simulink model "IFOR"  (Simulink 7.1)
settings: Solver=ode1  StartTime=0  StopTime=1  FixedStep=1e-5  MaxStep=1e-4  RelTol=1e-3  AbsTol=1e-6
undefined symbols (not defined in the file): I1, I2, I3, ids, Lm, P, P1, P2, P3, Rr, Rs, Tr, Ud, wb, Xlr, Xls, Xm
libraries: simulink x3
settings Model: Creator=Karsten  LastModifiedBy=Karsten  ExtModeTrigMode=oneshot  ExtModeArmWhenConnect=off
settings SolverCC: InitialStep=1e-4
settings DataIOCC: LimitDataPoints=off  SignalLoggingName=sigsOut
settings OptimizationCC: BooleanDataType=off  InlineInvariantSignals=on
settings DebuggingCC: SaveWithParameterizedLinksMsg=none  CheckExecutionContextPreStartOutputMsg=on  CheckExecutionContextRuntimeOutputMsg=on  SignalResolutionControl=TryResolveAllWithWarning  SolverPrmCheckMsg=none  MultiTaskDSMMsg=warning  MultiTaskCondExecSysMsg=none  StrictBusMsg=None
settings HardwareCC: TargetUnknown=on
settings RTWCC: TemplateMakefile=grt_vc.tmf  IncludeERTFirstTime=on
settings GRTTargetCC: TargetFcnLib=ansi_tfl_tmw.mat

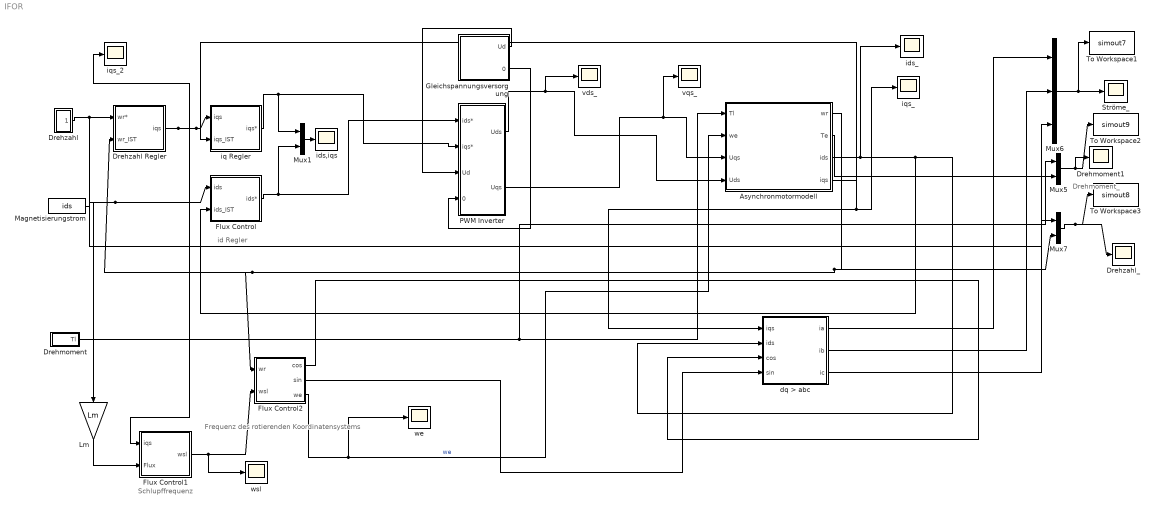
== system IFOR ==
  note: Schlupffrequenz
  note: Frequenz des rotierenden
      | Koordinatensystems
  note: id Regler
  note: Drehmoment_
  Asynchronmotormodell : Subsystem
  Drehmoment : Subsystem
  Drehmoment1 : Scope
      settings: TickLabels=on  TimeRange=0.001543443952852636  YMin=-3  YMax=6  DataFormat=Array  MaxDataPoints=500000
  Drehzahl : Subsystem
  Drehzahl Regler : Subsystem
  Drehzahl_ : Scope
      settings: TickLabels=on  TimeRange=0.5  YMin=156.4  YMax=157.1  DataFormat=Array  MaxDataPoints=500000
  Flux Control : Subsystem
  Flux Control1 : Subsystem
  Flux Control2 : Subsystem
  Gleichspannungsversorgung : Subsystem
  Lm : Gain  Orientation=down  Gain=Lm  ParameterDataType=sfix(16)  ParameterScaling=2^0  OutDataType=sfix(16)  OutScaling=2^0
  Magnetisierungstrom : Constant  Value=ids  OutDataType=sfix(16)  OutScaling=2^0
  Mux1 : Mux  Inputs=2
  Mux5 : Mux  Inputs=2
  Mux6 : Mux  Inputs=3
  Mux7 : Mux  Inputs=2
  PWM Inverter : Subsystem
  Ströme_ : Scope
      settings: TickLabels=on  TimeRange=0.008485639686684032  YMin=-4  YMax=4  DataFormat=Array  MaxDataPoints=500000
  To Workspace1 : ToWorkspace  VariableName=simout7  SampleTime=-1  SaveFormat=Structure
  To Workspace2 : ToWorkspace  VariableName=simout9  SampleTime=-1  SaveFormat=Structure
  To Workspace3 : ToWorkspace  VariableName=simout8  SampleTime=-1  SaveFormat=Structure
  dq > abc : Subsystem
  ids,iqs : Scope
      settings: TickLabels=on  TimeRange=0.5  YMin=-0.25  YMax=3  SaveName=ScopeData8  DataFormat=Array  MaxDataPoints=500000
  ids_ : Scope
      settings: TickLabels=on  TimeRange=0.3  YMin=0.65  YMax=0.8300000000000001  SaveName=ScopeData17  DataFormat=Array  MaxDataPoints=500000
  iq Regler : Subsystem
  iqs_ : Scope
      settings: TickLabels=on  TimeRange=0.3  YMin=3.15  YMax=3.8  SaveName=ScopeData18  DataFormat=Array  MaxDataPoints=500000
  iqs_2 : Scope
      settings: TickLabels=on  TimeRange=0.3  YMin=-1  YMax=-0.1  SaveName=ScopeData9  DataFormat=Array  MaxDataPoints=500000
  vds_ : Scope
      settings: TickLabels=on  TimeRange=0.3  YMin=-150  YMax=150  SaveName=ScopeData20  DataFormat=Array  MaxDataPoints=500000
  vqs_ : Scope
      settings: TickLabels=on  TimeRange=0.3  YMin=-200  YMax=200  SaveName=ScopeData19  DataFormat=Array  MaxDataPoints=500000
  we : Scope
      settings: TickLabels=on  YMin=31.4298  YMax=31.4301  SaveName=ScopeData3  DataFormat=Array  MaxDataPoints=500000
  wsl : Scope
      settings: TickLabels=on  TimeRange=0.5  YMin=-0.0225  YMax=0.0325  SaveName=ScopeData21  DataFormat=Array  MaxDataPoints=500000
  wires:
  Drehzahl/1(wr*) -> Drehzahl Regler/1(wr*), Mux7/1
  Flux Control2/3(we) -> we/1, Asynchronmotormodell/2(we)  "we"
  Mux6/1 -> Ströme_/1, To Workspace1/1
  Mux5/1 -> Drehmoment1/1, To Workspace2/1
  Mux7/1 -> Drehzahl_/1, To Workspace3/1
  PWM Inverter/2(Uqs) -> Asynchronmotormodell/3(Uqs), vqs_/1
  Asynchronmotormodell/4(iqs) -> dq > abc/1(iqs), iqs_/1, iq Regler/2(iqs_IST)
  Asynchronmotormodell/3(ids) -> ids_/1, dq > abc/2(ids), Flux Control/2(ids_IST)
  PWM Inverter/1(Uds) -> vds_/1, Asynchronmotormodell/4(Uds)
  Drehmoment/1(Tl) -> Asynchronmotormodell/1(Tl), Mux5/1
  Asynchronmotormodell/1(wr) -> Mux7/2, Drehzahl Regler/2(wr_IST), Flux Control2/1(wr)
  Asynchronmotormodell/2(Te) -> Mux5/2
  dq > abc/1(ia) -> Mux6/1
  dq > abc/2(ib) -> Mux6/2
  dq > abc/3(ic) -> Mux6/3
  iq Regler/1(iqs*) -> Mux1/1, PWM Inverter/2(iqs*)
  Drehzahl Regler/1(iqs) -> iq Regler/1(iqs), Flux Control1/1(iqs), iqs_2/1
  Flux Control/1(ids*) -> Mux1/2, PWM Inverter/1(ids*)
  Flux Control1/1(wsl) -> Flux Control2/2(wsl), wsl/1
  Flux Control2/1(cos) -> dq > abc/3(cos)
  Flux Control2/2(sin) -> dq > abc/4(sin)
  Magnetisierungstrom/1 -> Flux Control/1(ids), Lm/1
  Lm/1 -> Flux Control1/2(Flux)
  Gleichspannungsversorgung/2(0) -> PWM Inverter/4(0)
  Gleichspannungsversorgung/1(Ud) -> PWM Inverter/3(Ud)
  Mux1/1 -> ids,iqs/1

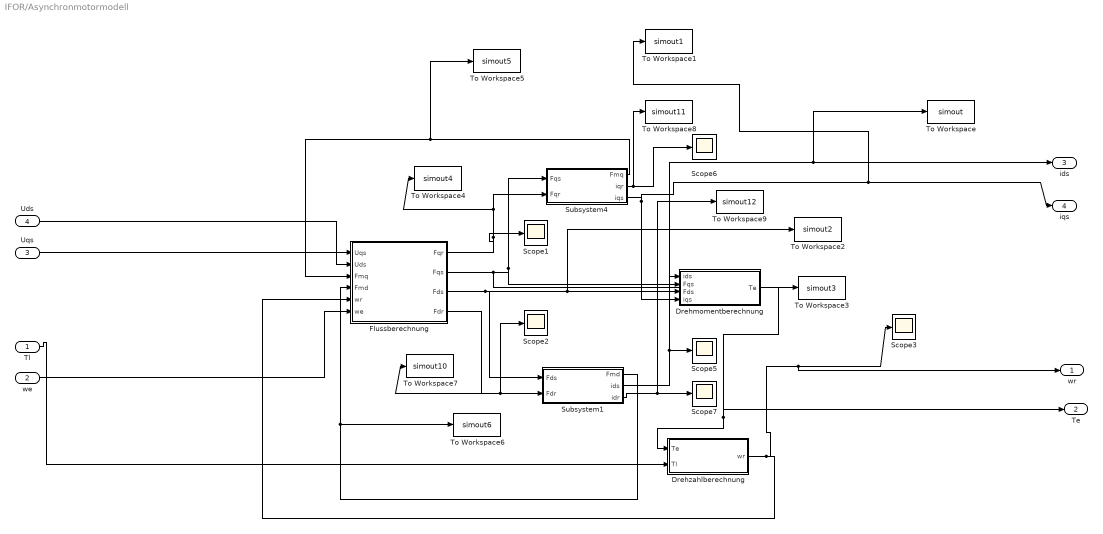
== system IFOR/Asynchronmotormodell ==
  Tl : Inport  OutDataType=sfix(16)  OutScaling=2^0
  we : Inport  Port=2  OutDataType=sfix(16)  OutScaling=2^0
  Uqs : Inport  Port=3  OutDataType=sfix(16)  OutScaling=2^0
  Uds : Inport  Port=4  OutDataType=sfix(16)  OutScaling=2^0
  Drehmomentberechnung : Subsystem
  Drehzahlberechnung : Subsystem
  Flussberechnung : Subsystem
  Scope{1..3,5..7} (6 alike) : Scope
      Scope1 settings: TimeRange=0.3  YMin=-47.25  YMax=-43.75  SaveName=ScopeData29
      Scope2 settings: TimeRange=0.3  YMin=386.5  YMax=393.5  SaveName=ScopeData30
      Scope3 settings: TimeRange=0.5  YMin=30  YMax=240  SaveName=Drehzahl1
      Scope5 settings: TimeRange=0.5  YMin=66.3  YMax=68.1  SaveName=ScopeData13
      Scope6 settings: TimeRange=0.3  YMin=-25  YMax=7.5  SaveName=ScopeData14
      Scope7 settings: TimeRange=1  YMin=-1  YMax=1  SaveName=ScopeData15
  Subsystem1 : Subsystem
  Subsystem4 : Subsystem
  To Workspace : ToWorkspace  VariableName=simout  SampleTime=-1  SaveFormat=Structure
  To Workspace1 : ToWorkspace  VariableName=simout1  SampleTime=-1  SaveFormat=Structure
  To Workspace2 : ToWorkspace  VariableName=simout2  SampleTime=-1  SaveFormat=Structure
  To Workspace3 : ToWorkspace  VariableName=simout3  SampleTime=-1  SaveFormat=Structure
  To Workspace4 : ToWorkspace  VariableName=simout4  SampleTime=-1  SaveFormat=Structure
  To Workspace5 : ToWorkspace  VariableName=simout5  SampleTime=-1  SaveFormat=Structure
  To Workspace6 : ToWorkspace  VariableName=simout6  SampleTime=-1  SaveFormat=Structure
  To Workspace7 : ToWorkspace  VariableName=simout10  SampleTime=-1  SaveFormat=Structure
  To Workspace8 : ToWorkspace  VariableName=simout11  SampleTime=-1  SaveFormat=Structure
  To Workspace9 : ToWorkspace  VariableName=simout12  SampleTime=-1  SaveFormat=Structure
  wr : Outport  OutDataType=sfix(16)  OutScaling=2^0
  Te : Outport  Port=2  OutDataType=sfix(16)  OutScaling=2^0
  ids : Outport  Port=3  OutDataType=sfix(16)  OutScaling=2^0
  iqs : Outport  Port=4  OutDataType=sfix(16)  OutScaling=2^0
  wires:
  Flussberechnung/1(Fqr) -> Subsystem4/2(Fqr), To Workspace4/1, Scope1/1
  Flussberechnung/2(Fqs) -> Subsystem4/1(Fqs), Drehmomentberechnung/2(Fqs), To Workspace3/1
  Subsystem4/1(Fmq) -> Flussberechnung/3(Fmq), To Workspace5/1
  Flussberechnung/3(Fds) -> Subsystem1/1(Fds), Drehmomentberechnung/3(Fds), To Workspace2/1
  Flussberechnung/4(Fdr) -> To Workspace7/1, Scope2/1, Subsystem1/2(Fdr)
  Subsystem1/1(Fmd) -> Flussberechnung/4(Fmd), To Workspace6/1
  Subsystem1/2(ids) -> Drehmomentberechnung/1(ids), Scope5/1, ids/1, To Workspace/1
  Subsystem1/3(idr) -> Scope7/1, To Workspace9/1
  Subsystem4/3(iqs) -> Drehmomentberechnung/4(iqs), iqs/1, To Workspace1/1
  Drehmomentberechnung/1(Te) -> Drehzahlberechnung/1(Te), Te/1
  Drehzahlberechnung/1(wr) -> Flussberechnung/5(wr), Scope3/1, wr/1
  Tl/1 -> Drehzahlberechnung/2(Tl)
  Subsystem4/2(iqr) -> Scope6/1, To Workspace8/1
  we/1 -> Flussberechnung/6(we)
  Uqs/1 -> Flussberechnung/1(Uqs)
  Uds/1 -> Flussberechnung/2(Uds)

== system IFOR/Drehmoment ==
  Step2 : Step  Time=.2  After=3  SampleTime=0
  Step3 : Step  Time=0.05  After=0  SampleTime=0
  Step4 : Step  Time=30  After=0  SampleTime=0
  Sum1 : Sum  Inputs=|+++  OutDataType=sfix(16)  OutScaling=2^0  SaturateOnIntegerOverflow=on  InputSameDT=on  OutDataTypeStr=Inherit: Same as first input
  Tl : Outport  OutDataType=sfix(16)  OutScaling=2^0
  wires:
  Step3/1 -> Sum1/2
  Step2/1 -> Sum1/1
  Step4/1 -> Sum1/3
  Sum1/1 -> Tl/1

== system IFOR/Drehzahl ==
  Magnetisierungstrom : Constant  Value=wb/5  OutDataType=sfix(16)  OutScaling=2^0
  Repeating Sequence : simulink/Sources/Repeating Sequence  SystemSampleTime=-1  rep_seq_t=[0 .15 .25 .4 .55 .6 10]  rep_seq_y=[0 .5*wb .5*wb .2*wb .2*wb .4*wb .2*wb]
  Repeating Sequence1 : simulink/Sources/Repeating Sequence  SystemSampleTime=-1  rep_seq_t=[0 .15 .25 .4 .55 .6 10]  rep_seq_y=[0 .5*wb .5*wb .5*wb .5*wb .2*wb .2*wb]
  wr* : Outport  OutDataType=sfix(16)  OutScaling=2^0
  wires:
  Repeating Sequence1/1 -> wr*/1

== system IFOR/Drehzahl Regler ==
  wr* : Inport  OutDataType=sfix(16)  OutScaling=2^0
  wr_IST : Inport  Port=2  OutDataType=sfix(16)  OutScaling=2^0
  Gain1 : Gain  Gain=P1  ParameterDataType=sfix(16)  ParameterScaling=2^0  OutDataType=sfix(16)  OutScaling=2^0
  Gain2 : Gain  Gain=I1  ParameterDataType=sfix(16)  ParameterScaling=2^0  OutDataType=sfix(16)  OutScaling=2^0
  Integrator : Integrator
  Sum4 : Sum  Inputs=|++  OutDataType=sfix(16)  OutScaling=2^0
  Sum5 : Sum  Inputs=|+-  OutDataType=sfix(16)  OutScaling=2^0
  ia4 : Scope
      settings: TickLabels=on  YMin=2675  YMax=3100  SaveName=ScopeData5  DataFormat=Array  MaxDataPoints=500000
  iqs : Outport  OutDataType=sfix(16)  OutScaling=2^0  InitialOutput=0
  wires:
  wr*/1 -> Sum5/1
  Integrator/1 -> Sum4/2
  Gain1/1 -> Sum4/1
  Gain2/1 -> Integrator/1
  Sum5/1 -> Gain1/1, Gain2/1
  wr_IST/1 -> Sum5/2
  Sum4/1 -> ia4/1, iqs/1

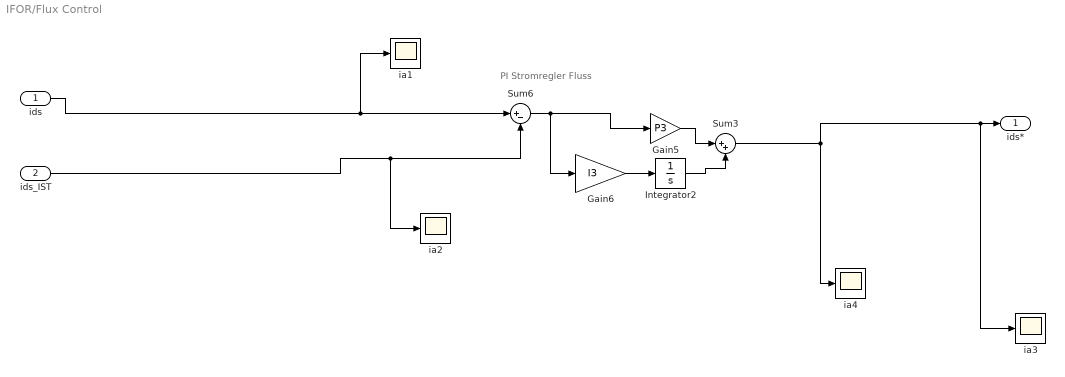
== system IFOR/Flux Control ==
  note: PI Stromregler Fluss
  ids : Inport  OutDataType=sfix(16)  OutScaling=2^0
  ids_IST : Inport  Port=2  OutDataType=sfix(16)  OutScaling=2^0
  Gain5 : Gain  Gain=P3  ParameterDataType=sfix(16)  ParameterScaling=2^0  OutDataType=sfix(16)  OutScaling=2^0
  Gain6 : Gain  Gain=I3  ParameterDataType=sfix(16)  ParameterScaling=2^0  OutDataType=sfix(16)  OutScaling=2^0
  Integrator2 : Integrator
  Sum3 : Sum  Inputs=|++  OutDataType=sfix(16)  OutScaling=2^0
  Sum6 : Sum  Inputs=|+-  OutDataType=sfix(16)  OutScaling=2^0
  ia{1..4} (4 alike) : Scope
      ia1 settings: TickLabels=on  YMin=2.3  YMax=2.3  SaveName=ScopeData24  DataFormat=Array  MaxDataPoints=500000
      ia2 settings: TickLabels=on  YMin=0.685  YMax=0.745  SaveName=ScopeData25  DataFormat=Array  MaxDataPoints=500000
      ia3 settings: TickLabels=on  YMin=-0.05  YMax=1  SaveName=ScopeData26  DataFormat=Array  MaxDataPoints=500000
      ia4 settings: TickLabels=on  YMin=-0.25  SaveName=ScopeData6  DataFormat=Array  MaxDataPoints=500000
  ids* : Outport  OutDataType=sfix(16)  OutScaling=2^0  InitialOutput=0
  wires:
  Integrator2/1 -> Sum3/2
  Gain5/1 -> Sum3/1
  Gain6/1 -> Integrator2/1
  Sum6/1 -> Gain5/1, Gain6/1
  ids_IST/1 -> Sum6/2, ia2/1
  Sum3/1 -> ia4/1, ids*/1, ia3/1
  ids/1 -> Sum6/1, ia1/1

== system IFOR/Flux Control1 ==
  iqs : Inport  OutDataType=sfix(16)  OutScaling=2^0
  Flux : Inport  Port=2  OutDataType=sfix(16)  OutScaling=2^0
  Gain : Gain  Gain=Lm/(Tr)  ParameterDataType=sfix(16)  ParameterScaling=2^0  OutDataType=sfix(16)  OutScaling=2^0  SaturateOnIntegerOverflow=on  OutDataTypeStr=Inherit: Same as input  ParamDataTypeStr=Inherit: Same as input
  Product : Product  OutDataType=sfix(16)  OutScaling=2^0  SaturateOnIntegerOverflow=on  InputSameDT=on  OutDataTypeStr=Inherit: Same as first input
  wsl : Outport  OutDataType=sfix(16)  OutScaling=2^0  InitialOutput=0
  wires:
  iqs/1 -> Gain/1
  Product/1 -> wsl/1
  Gain/1 -> Product/1
  Flux/1 -> Product/2

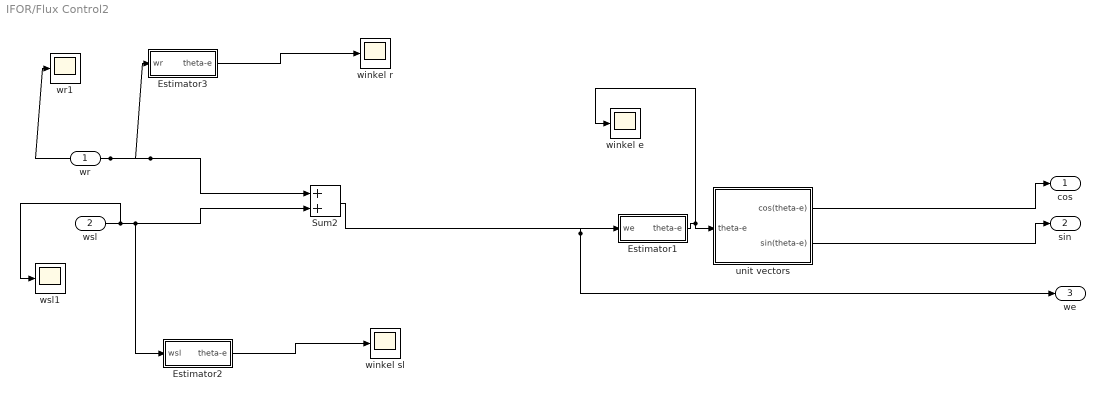
== system IFOR/Flux Control2 ==
  wr : Inport  OutDataType=sfix(16)  OutScaling=2^0
  wsl : Inport  Port=2  OutDataType=sfix(16)  OutScaling=2^0
  Estimator1 : Subsystem
  Estimator2 : Subsystem
  Estimator3 : Subsystem
  Sum2 : Sum  OutDataType=sfix(16)  OutScaling=2^0  SaturateOnIntegerOverflow=on  InputSameDT=on  OutDataTypeStr=Inherit: Same as first input
  unit vectors : Subsystem
  winkel e : Scope
      settings: TickLabels=on  YMin=0  YMax=6.5  SaveName=ScopeData4  DataFormat=Array  MaxDataPoints=500000
  winkel r : Scope
      settings: TickLabels=on  TimeRange=0.5  YMin=0  YMax=6.5  SaveName=ScopeData11  DataFormat=Array  MaxDataPoints=500000
  winkel sl : Scope
      settings: TickLabels=on  TimeRange=0.5  YMin=1.69116  YMax=1.69132  SaveName=ScopeData10  DataFormat=Array  MaxDataPoints=500000
  wr1 : Scope
      settings: TickLabels=on  YMin=156  YMax=170  SaveName=ScopeData12  DataFormat=Array  MaxDataPoints=500000
  wsl1 : Scope
      settings: TickLabels=on  YMin=-0.175  YMax=0.225  SaveName=ScopeData16  DataFormat=Array  MaxDataPoints=500000
  cos : Outport  OutDataType=sfix(16)  OutScaling=2^0  InitialOutput=0
  sin : Outport  Port=2  OutDataType=sfix(16)  OutScaling=2^0  InitialOutput=0
  we : Outport  Port=3  OutDataType=sfix(16)  OutScaling=2^0  InitialOutput=0
  wires:
  wr/1 -> Sum2/1, Estimator3/1(wr), wr1/1
  wsl/1 -> Sum2/2, Estimator2/1(wsl), wsl1/1
  unit vectors/1(cos(theta-e)) -> cos/1
  unit vectors/2(sin(theta-e)) -> sin/1
  Estimator1/1(theta-e) -> unit vectors/1(theta-e), winkel e/1
  Sum2/1 -> we/1, Estimator1/1(we)
  Estimator2/1(theta-e) -> winkel sl/1
  Estimator3/1(theta-e) -> winkel r/1

== system IFOR/Gleichspannungsversorgung ==
  Constant4 : Constant  Value=0  OutDataType=sfix(16)  OutScaling=2^0
  Constant5 : Constant  Value=Ud  OutDataType=sfix(16)  OutScaling=2^0
  Ud : Outport  OutDataType=sfix(16)  OutScaling=2^0  InitialOutput=0
  0 : Outport  Port=2  OutDataType=sfix(16)  OutScaling=2^0  InitialOutput=0
  wires:
  Constant4/1 -> 0/1
  Constant5/1 -> Ud/1

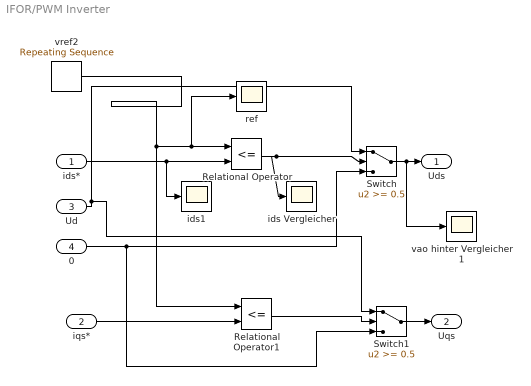
== system IFOR/PWM Inverter ==
  ids* : Inport  OutDataType=sfix(16)  OutScaling=2^0
  iqs* : Inport  Port=2  OutDataType=sfix(16)  OutScaling=2^0
  Ud : Inport  Port=3  OutDataType=sfix(16)  OutScaling=2^0
  0 : Inport  Port=4  OutDataType=sfix(16)  OutScaling=2^0
  Relational Operator : RelationalOperator  Operator=<=  InputSameDT=on
  Relational Operator1 : RelationalOperator  Operator=<=  InputSameDT=on
  Switch : Switch  Threshold=0.5  SaturateOnIntegerOverflow=on  InputSameDT=on
  Switch1 : Switch  Threshold=0.5  SaturateOnIntegerOverflow=on  InputSameDT=on
  ids Vergleicher : Scope
      settings: TickLabels=on  TimeRange=8.811583259921477e-005  YMin=-1  YMax=1  SaveName=ScopeData35  DataFormat=Array  MaxDataPoints=500000
  ids1 : Scope
      settings: TickLabels=on  TimeRange=0.3  YMin=-0.55  YMax=0.15  SaveName=ScopeData34  DataFormat=Array  MaxDataPoints=500000
  ref : Scope
      settings: TickLabels=on  TimeRange=0.3  YMin=0.9999999998750002  YMax=1.000000000125  SaveName=ScopeData33  DataFormat=Array  MaxDataPoints=500000
  vao hinter Vergleicher1 : Scope
      settings: TickLabels=on  TimeRange=0.3  YMin=-2  YMax=2  SaveName=ScopeData36  DataFormat=Array  MaxDataPoints=500000
  vref2 : simulink/Sources/Repeating Sequence  SystemSampleTime=-1  rep_seq_t=[0 25e-9 50e-9 75e-9 100e-9]  rep_seq_y=[0 1 0 -1 0]
  Uds : Outport  OutDataType=sfix(16)  OutScaling=2^0
  Uqs : Outport  Port=2  OutDataType=sfix(16)  OutScaling=2^0
  wires:
  ids*/1 -> Relational Operator/2, ids1/1
  Switch/1 -> Uds/1, vao hinter Vergleicher1/1
  Ud/1 -> Switch/1, Switch1/1
  Relational Operator/1 -> Switch/2, ids Vergleicher/1
  iqs*/1 -> Relational Operator1/2
  Switch1/1 -> Uqs/1
  Relational Operator1/1 -> Switch1/2
  vref2/1 -> Relational Operator/1, ref/1, Relational Operator1/1
  0/1 -> Switch/3, Switch1/3

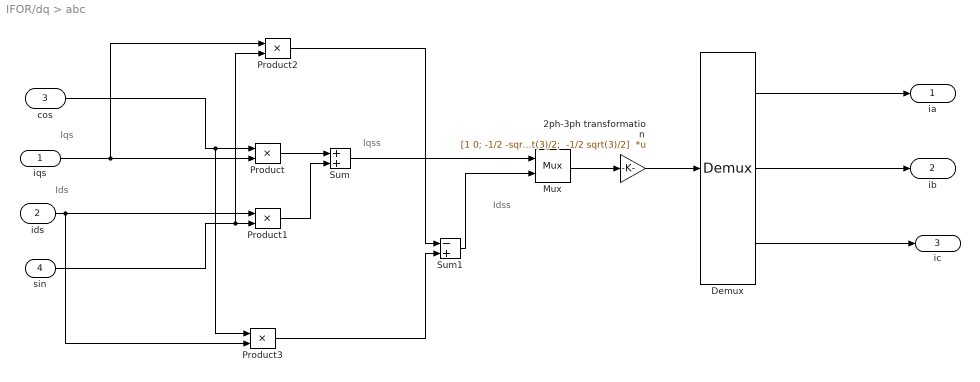
== system IFOR/dq > abc ==
  note: Ids
  note: Idss
  note: Iqs
  note: Iqss
  iqs : Inport  OutDataType=sfix(16)  OutScaling=2^0
  ids : Inport  Port=2  OutDataType=sfix(16)  OutScaling=2^0
  cos : Inport  Port=3  OutDataType=sfix(16)  OutScaling=2^0
  sin : Inport  Port=4  OutDataType=sfix(16)  OutScaling=2^0
  2ph-3ph transformation : Gain  Gain="[1 0; -1/2 -sqrt(3)/2;  -1/2 sqrt(3)/2]"  Multiplication=Matrix(K*u)  ParameterDataType=sfix(16)  ParameterScaling=2^0  OutDataType=sfix(16)  OutScaling=2^0  SaturateOnIntegerOverflow=on  OutDataTypeStr=Inherit: Same as input  ParamDataTypeStr=Inherit: Same as input
  Demux : Demux  Outputs=3
  Mux : Mux  Inputs=2
  Product{,1..3} (4 alike) : Product  OutDataType=sfix(16)  OutScaling=2^0  SaturateOnIntegerOverflow=on  InputSameDT=on  OutDataTypeStr=Inherit: Same as first input
  Sum : Sum  OutDataType=sfix(16)  OutScaling=2^0  SaturateOnIntegerOverflow=on  InputSameDT=on  OutDataTypeStr=Inherit: Same as first input
  Sum1 : Sum  Inputs=-+  OutDataType=sfix(16)  OutScaling=2^0  SaturateOnIntegerOverflow=on  InputSameDT=on  OutDataTypeStr=Inherit: Same as first input
  ia : Outport  OutDataType=sfix(16)  OutScaling=2^0
  ib : Outport  Port=2  OutDataType=sfix(16)  OutScaling=2^0
  ic : Outport  Port=3  OutDataType=sfix(16)  OutScaling=2^0
  wires:
  Demux/3 -> ic/1
  Demux/2 -> ib/1
  Demux/1 -> ia/1
  iqs/1 -> Product/2, Product2/1
  ids/1 -> Product1/1, Product3/2
  Mux/1 -> 2ph-3ph transformation/1
  Product2/1 -> Sum1/1
  Product3/1 -> Sum1/2
  cos/1 -> Product/1, Product3/1
  sin/1 -> Product1/2, Product2/2
  Product1/1 -> Sum/2
  Product/1 -> Sum/1
  Sum/1 -> Mux/1
  Sum1/1 -> Mux/2
  2ph-3ph transformation/1 -> Demux/1

== system IFOR/iq Regler ==
  note: PI Stromregler Drehmoment
  iqs : Inport  OutDataType=sfix(16)  OutScaling=2^0
  iqs_IST : Inport  Port=2  OutDataType=sfix(16)  OutScaling=2^0
  Gain3 : Gain  Gain=P2  ParameterDataType=sfix(16)  ParameterScaling=2^0  OutDataType=sfix(16)  OutScaling=2^0
  Gain4 : Gain  Gain=I2  ParameterDataType=sfix(16)  ParameterScaling=2^0  OutDataType=sfix(16)  OutScaling=2^0
  Integrator1 : Integrator
  Sum1 : Sum  Inputs=|++  OutDataType=sfix(16)  OutScaling=2^0
  Sum2 : Sum  Inputs=|+-  OutDataType=sfix(16)  OutScaling=2^0
  ia1 : Scope
      settings: TickLabels=on  YMin=-100  YMax=100  SaveName=ScopeData22  DataFormat=Array  MaxDataPoints=500000
  ia2 : Scope
      settings: TickLabels=on  YMin=-100  YMax=100  SaveName=ScopeData23  DataFormat=Array  MaxDataPoints=500000
  ia4 : Scope
      settings: TickLabels=on  YMin=0.275  YMax=0.825  SaveName=ScopeData7  DataFormat=Array  MaxDataPoints=500000
  iqs* : Outport  OutDataType=sfix(16)  OutScaling=2^0  InitialOutput=0
  wires:
  iqs_IST/1 -> Sum2/2, ia2/1
  Sum1/1 -> ia4/1, iqs*/1, ia1/1
  Sum2/1 -> Gain4/1, Gain3/1
  Gain4/1 -> Integrator1/1
  Gain3/1 -> Sum1/1
  Integrator1/1 -> Sum1/2
  iqs/1 -> Sum2/1

== system IFOR/Asynchronmotormodell/Drehmomentberechnung ==
  ids : Inport  OutDataType=sfix(16)  OutScaling=2^0
  Fqs : Inport  Port=2  OutDataType=sfix(16)  OutScaling=2^0
  Fds : Inport  Port=3  OutDataType=sfix(16)  OutScaling=2^0
  iqs : Inport  Port=4  OutDataType=sfix(16)  OutScaling=2^0
  1.5*P/(2*wb) : Gain  Gain=1.5*P/(2*wb)  ParameterDataType=sfix(16)  ParameterScaling=2^0  OutDataType=sfix(16)  OutScaling=2^0
  Add3 : Sum  Inputs=-+  OutDataType=sfix(16)  OutScaling=2^-10
  Product1 : Product  OutDataType=sfix(16)  OutScaling=2^0  RndMeth=Zero
  Product2 : Product  OutDataType=sfix(16)  OutScaling=2^0  RndMeth=Zero
  Te : Outport  OutDataType=sfix(16)  OutScaling=2^0
  wires:
  Product1/1 -> Add3/1
  Product2/1 -> Add3/2
  Add3/1 -> 1.5*P/(2*wb)/1
  1.5*P/(2*wb)/1 -> Te/1
  ids/1 -> Product1/1
  Fqs/1 -> Product1/2
  Fds/1 -> Product2/1
  iqs/1 -> Product2/2

== system IFOR/Asynchronmotormodell/Drehzahlberechnung ==
  Te : Inport  OutDataType=sfix(16)  OutScaling=2^0
  Tl : Inport  Port=2  OutDataType=sfix(16)  OutScaling=2^0
  Add3 : Sum  Inputs=+-  OutDataType=sfix(16)  OutScaling=2^-10
  Integrator : Integrator
  P/(2*J) : Gain  Gain=P/(2*0.006)  ParameterDataType=sfix(16)  ParameterScaling=2^0  OutDataType=sfix(16)  OutScaling=2^0
  wr : Outport  OutDataType=sfix(16)  OutScaling=2^0
  wires:
  Te/1 -> Add3/1
  Tl/1 -> Add3/2
  Add3/1 -> P/(2*J)/1
  P/(2*J)/1 -> Integrator/1
  Integrator/1 -> wr/1

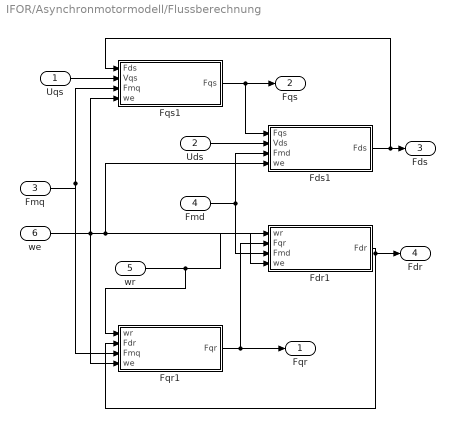
== system IFOR/Asynchronmotormodell/Flussberechnung ==
  Uqs : Inport  OutDataType=sfix(16)  OutScaling=2^0
  Uds : Inport  Port=2  OutDataType=sfix(16)  OutScaling=2^0
  Fmq : Inport  Port=3  OutDataType=sfix(16)  OutScaling=2^0
  Fmd : Inport  Port=4  OutDataType=sfix(16)  OutScaling=2^0
  wr : Inport  Port=5  OutDataType=sfix(16)  OutScaling=2^0
  we : Inport  Port=6  OutDataType=sfix(16)  OutScaling=2^0
  Fdr1 : Subsystem
  Fds1 : Subsystem
  Fqr1 : Subsystem
  Fqs1 : Subsystem
  Fqr : Outport  OutDataType=sfix(16)  OutScaling=2^0
  Fqs : Outport  Port=2  OutDataType=sfix(16)  OutScaling=2^0
  Fds : Outport  Port=3  OutDataType=sfix(16)  OutScaling=2^0
  Fdr : Outport  Port=4  OutDataType=sfix(16)  OutScaling=2^0
  wires:
  Uqs/1 -> Fqs1/2(Vqs)
  Fqs1/1(Fqs) -> Fqs/1, Fds1/1(Fqs)
  Uds/1 -> Fds1/2(Vds)
  Fmd/1 -> Fds1/3(Fmd), Fdr1/3(Fmd)
  wr/1 -> Fdr1/1(wr), Fqr1/1(wr)
  Fmq/1 -> Fqs1/3(Fmq), Fqr1/3(Fmq)
  Fdr1/1(Fdr) -> Fqr1/2(Fdr), Fdr/1
  Fqr1/1(Fqr) -> Fqr/1, Fdr1/2(Fqr)
  Fds1/1(Fds) -> Fds/1, Fqs1/1(Fds)
  we/1 -> Fqr1/4(we), Fqs1/4(we), Fdr1/4(we), Fds1/4(we)

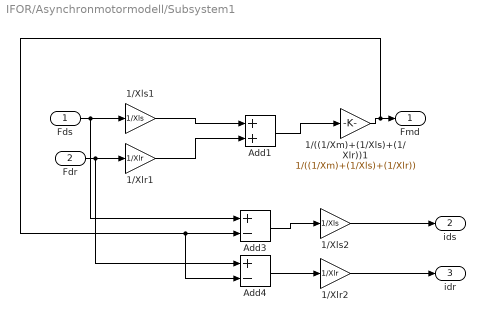
== system IFOR/Asynchronmotormodell/Subsystem1 ==
  Fds : Inport  OutDataType=sfix(16)  OutScaling=2^0
  Fdr : Inport  Port=2  OutDataType=sfix(16)  OutScaling=2^0
  1/((1/Xm)+(1/Xls)+(1/Xlr))1 : Gain  Gain=1/((1/Xm)+(1/Xls)+(1/Xlr))  ParameterDataType=sfix(16)  ParameterScaling=2^0  OutDataType=sfix(16)  OutScaling=2^0
  1/Xlr1 : Gain  Gain=1/Xlr  ParameterDataType=sfix(16)  ParameterScaling=2^0  OutDataType=sfix(16)  OutScaling=2^0
  1/Xlr2 : Gain  Gain=1/Xlr  ParameterDataType=sfix(16)  ParameterScaling=2^0  OutDataType=sfix(16)  OutScaling=2^0
  1/Xls1 : Gain  Gain=1/Xls  ParameterDataType=sfix(16)  ParameterScaling=2^0  OutDataType=sfix(16)  OutScaling=2^0
  1/Xls2 : Gain  Gain=1/Xls  ParameterDataType=sfix(16)  ParameterScaling=2^0  OutDataType=sfix(16)  OutScaling=2^0
  Add1 : Sum  OutDataType=sfix(16)  OutScaling=2^-10
  Add3 : Sum  Inputs=+-  OutDataType=sfix(16)  OutScaling=2^-10
  Add4 : Sum  Inputs=+-  OutDataType=sfix(16)  OutScaling=2^-10
  Fmd : Outport  OutDataType=sfix(16)  OutScaling=2^0
  ids : Outport  Port=2  OutDataType=sfix(16)  OutScaling=2^0
  idr : Outport  Port=3  OutDataType=sfix(16)  OutScaling=2^0
  wires:
  Fds/1 -> 1/Xls1/1, Add3/1
  Fdr/1 -> 1/Xlr1/1, Add4/1
  1/Xls1/1 -> Add1/1
  1/Xlr1/1 -> Add1/2
  Add1/1 -> 1/((1/Xm)+(1/Xls)+(1/Xlr))1/1
  1/((1/Xm)+(1/Xls)+(1/Xlr))1/1 -> Fmd/1, Add3/2, Add4/2
  Add3/1 -> 1/Xls2/1
  Add4/1 -> 1/Xlr2/1
  1/Xlr2/1 -> idr/1
  1/Xls2/1 -> ids/1

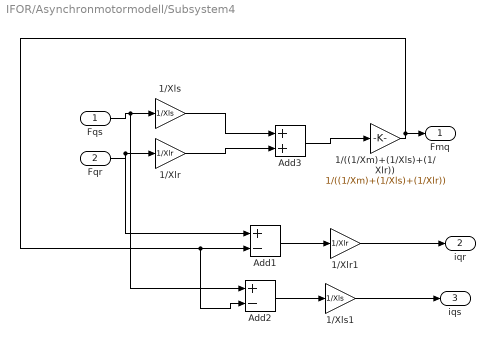
== system IFOR/Asynchronmotormodell/Subsystem4 ==
  Fqs : Inport  OutDataType=sfix(16)  OutScaling=2^0
  Fqr : Inport  Port=2  OutDataType=sfix(16)  OutScaling=2^0
  1/((1/Xm)+(1/Xls)+(1/Xlr)) : Gain  Gain=1/((1/Xm)+(1/Xls)+(1/Xlr))  ParameterDataType=sfix(16)  ParameterScaling=2^0  OutDataType=sfix(16)  OutScaling=2^0
  1/Xlr : Gain  Gain=1/Xlr  ParameterDataType=sfix(16)  ParameterScaling=2^0  OutDataType=sfix(16)  OutScaling=2^0
  1/Xlr1 : Gain  Gain=1/Xlr  ParameterDataType=sfix(16)  ParameterScaling=2^0  OutDataType=sfix(16)  OutScaling=2^0
  1/Xls : Gain  Gain=1/Xls  ParameterDataType=sfix(16)  ParameterScaling=2^0  OutDataType=sfix(16)  OutScaling=2^0
  1/Xls1 : Gain  Gain=1/Xls  ParameterDataType=sfix(16)  ParameterScaling=2^0  OutDataType=sfix(16)  OutScaling=2^0
  Add1 : Sum  Inputs=+-  OutDataType=sfix(16)  OutScaling=2^-10
  Add2 : Sum  Inputs=+-  OutDataType=sfix(16)  OutScaling=2^-10
  Add3 : Sum  OutDataType=sfix(16)  OutScaling=2^-10
  Fmq : Outport  OutDataType=sfix(16)  OutScaling=2^0
  iqr : Outport  Port=2  OutDataType=sfix(16)  OutScaling=2^0
  iqs : Outport  Port=3  OutDataType=sfix(16)  OutScaling=2^0
  wires:
  Fqs/1 -> 1/Xls/1, Add2/1
  Fqr/1 -> 1/Xlr/1, Add1/1
  1/Xls/1 -> Add3/1
  1/Xlr/1 -> Add3/2
  Add3/1 -> 1/((1/Xm)+(1/Xls)+(1/Xlr))/1
  1/((1/Xm)+(1/Xls)+(1/Xlr))/1 -> Fmq/1, Add1/2, Add2/2
  Add1/1 -> 1/Xlr1/1
  1/Xlr1/1 -> iqr/1
  Add2/1 -> 1/Xls1/1
  1/Xls1/1 -> iqs/1

== system IFOR/Flux Control2/Estimator1 ==
  we : Inport  OutDataType=sfix(16)  OutScaling=2^0
  Constant : Constant  Value=2*pi  OutDataType=sfix(16)  OutScaling=2^0
  Integrator : Integrator  InitialCondition=pi/6
  Math Function3 : Math  Operator=mod  OutDataType=sfix(16)  OutScaling=2^0  SaturateOnIntegerOverflow=on
  theta-e : Outport  OutDataType=sfix(16)  OutScaling=2^0
  wires:
  Math Function3/1 -> theta-e/1
  Integrator/1 -> Math Function3/1
  Constant/1 -> Math Function3/2
  we/1 -> Integrator/1

== system IFOR/Flux Control2/Estimator2 ==
  wsl : Inport  OutDataType=sfix(16)  OutScaling=2^0
  Constant : Constant  Value=2*pi  OutDataType=sfix(16)  OutScaling=2^0
  Integrator : Integrator  InitialCondition=pi/6
  Math Function3 : Math  Operator=mod  OutDataType=sfix(16)  OutScaling=2^0  SaturateOnIntegerOverflow=on
  theta-e : Outport  OutDataType=sfix(16)  OutScaling=2^0
  wires:
  wsl/1 -> Integrator/1
  Constant/1 -> Math Function3/2
  Integrator/1 -> Math Function3/1
  Math Function3/1 -> theta-e/1

== system IFOR/Flux Control2/Estimator3 ==
  wr : Inport  OutDataType=sfix(16)  OutScaling=2^0
  Constant : Constant  Value=2*pi  OutDataType=sfix(16)  OutScaling=2^0
  Integrator : Integrator  InitialCondition=pi/6
  Math Function3 : Math  Operator=mod  OutDataType=sfix(16)  OutScaling=2^0  SaturateOnIntegerOverflow=on
  theta-e : Outport  OutDataType=sfix(16)  OutScaling=2^0
  wires:
  wr/1 -> Integrator/1
  Constant/1 -> Math Function3/2
  Integrator/1 -> Math Function3/1
  Math Function3/1 -> theta-e/1

== system IFOR/Flux Control2/unit vectors ==
  theta-e : Inport  OutDataType=sfix(16)  OutScaling=2^0
  Trigonometric Function : Trigonometry
  Trigonometric Function1 : Trigonometry  Operator=cos
  cos(theta-e) : Outport  OutDataType=sfix(16)  OutScaling=2^0
  sin(theta-e) : Outport  Port=2  OutDataType=sfix(16)  OutScaling=2^0
  wires:
  Trigonometric Function/1 -> sin(theta-e)/1
  Trigonometric Function1/1 -> cos(theta-e)/1
  theta-e/1 -> Trigonometric Function1/1, Trigonometric Function/1

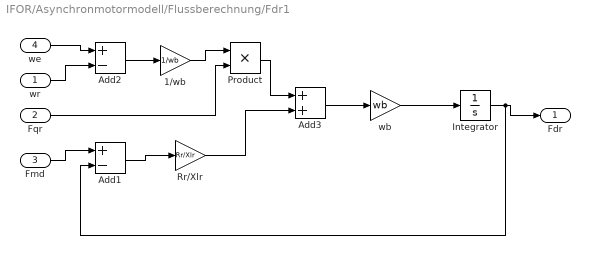
== system IFOR/Asynchronmotormodell/Flussberechnung/Fdr1 ==
  wr : Inport  OutDataType=sfix(16)  OutScaling=2^0
  Fqr : Inport  Port=2  OutDataType=sfix(16)  OutScaling=2^0
  Fmd : Inport  Port=3  OutDataType=sfix(16)  OutScaling=2^0
  we : Inport  Port=4  OutDataType=sfix(16)  OutScaling=2^0
  1/wb : Gain  Gain=1/wb  ParameterDataType=sfix(16)  ParameterScaling=2^0  OutDataType=sfix(16)  OutScaling=2^0
  Add1 : Sum  Inputs=+-  OutDataType=sfix(16)  OutScaling=2^-10
  Add2 : Sum  Inputs=+-  OutDataType=sfix(16)  OutScaling=2^-10
  Add3 : Sum  OutDataType=sfix(16)  OutScaling=2^-10
  Integrator : Integrator
  Product : Product  OutDataType=sfix(16)  OutScaling=2^0  RndMeth=Zero
  Rr/Xlr : Gain  Gain=Rr/Xlr  ParameterDataType=sfix(16)  ParameterScaling=2^0  OutDataType=sfix(16)  OutScaling=2^0
  wb : Gain  Gain=wb  ParameterDataType=sfix(16)  ParameterScaling=2^0  OutDataType=sfix(16)  OutScaling=2^0
  Fdr : Outport  OutDataType=sfix(16)  OutScaling=2^0
  wires:
  wr/1 -> Add2/2
  Fqr/1 -> Product/2
  1/wb/1 -> Product/1
  Add2/1 -> 1/wb/1
  Fmd/1 -> Add1/1
  Add1/1 -> Rr/Xlr/1
  Rr/Xlr/1 -> Add3/2
  Product/1 -> Add3/1
  Add3/1 -> wb/1
  wb/1 -> Integrator/1
  Integrator/1 -> Fdr/1, Add1/2
  we/1 -> Add2/1

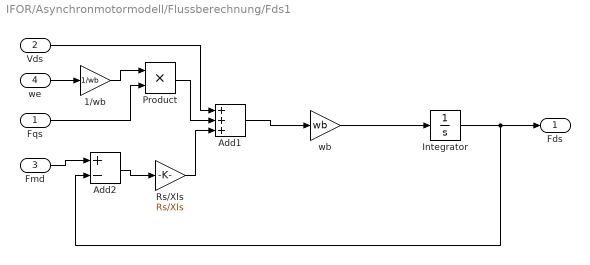
== system IFOR/Asynchronmotormodell/Flussberechnung/Fds1 ==
  Fqs : Inport  OutDataType=sfix(16)  OutScaling=2^0
  Vds : Inport  Port=2  OutDataType=sfix(16)  OutScaling=2^0
  Fmd : Inport  Port=3  OutDataType=sfix(16)  OutScaling=2^0
  we : Inport  Port=4  OutDataType=sfix(16)  OutScaling=2^0
  1/wb : Gain  Gain=1/wb  ParameterDataType=sfix(16)  ParameterScaling=2^0  OutDataType=sfix(16)  OutScaling=2^0
  Add1 : Sum  Inputs=+++  OutDataType=sfix(16)  OutScaling=2^-10
  Add2 : Sum  Inputs=+-  OutDataType=sfix(16)  OutScaling=2^-10
  Integrator : Integrator
  Product : Product  OutDataType=sfix(16)  OutScaling=2^0  RndMeth=Zero
  Rs/Xls : Gain  Gain=Rs/Xls  ParameterDataType=sfix(16)  ParameterScaling=2^0  OutDataType=sfix(16)  OutScaling=2^0
  wb : Gain  Gain=wb  ParameterDataType=sfix(16)  ParameterScaling=2^0  OutDataType=sfix(16)  OutScaling=2^0
  Fds : Outport  OutDataType=sfix(16)  OutScaling=2^0
  wires:
  we/1 -> 1/wb/1
  1/wb/1 -> Product/1
  Fqs/1 -> Product/2
  Product/1 -> Add1/2
  Vds/1 -> Add1/1
  Fmd/1 -> Add2/1
  Add2/1 -> Rs/Xls/1
  Rs/Xls/1 -> Add1/3
  Add1/1 -> wb/1
  wb/1 -> Integrator/1
  Integrator/1 -> Fds/1, Add2/2

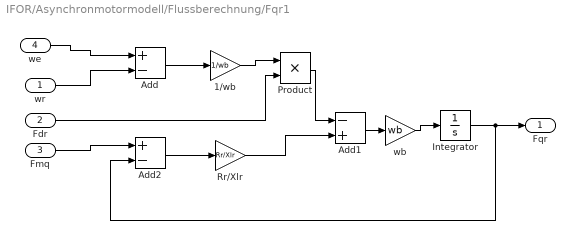
== system IFOR/Asynchronmotormodell/Flussberechnung/Fqr1 ==
  wr : Inport  OutDataType=sfix(16)  OutScaling=2^0
  Fdr : Inport  Port=2  OutDataType=sfix(16)  OutScaling=2^0
  Fmq : Inport  Port=3  OutDataType=sfix(16)  OutScaling=2^0
  we : Inport  Port=4  OutDataType=sfix(16)  OutScaling=2^0
  1/wb : Gain  Gain=1/wb  ParameterDataType=sfix(16)  ParameterScaling=2^0  OutDataType=sfix(16)  OutScaling=2^0
  Add : Sum  Inputs=+-  OutDataType=sfix(16)  OutScaling=2^-10
  Add1 : Sum  Inputs=-+  OutDataType=sfix(16)  OutScaling=2^-10
  Add2 : Sum  Inputs=+-  OutDataType=sfix(16)  OutScaling=2^-10
  Integrator : Integrator
  Product : Product  OutDataType=sfix(16)  OutScaling=2^0  RndMeth=Zero
  Rr/Xlr : Gain  Gain=Rr/Xlr  ParameterDataType=sfix(16)  ParameterScaling=2^0  OutDataType=sfix(16)  OutScaling=2^0
  wb : Gain  Gain=wb  ParameterDataType=sfix(16)  ParameterScaling=2^0  OutDataType=sfix(16)  OutScaling=2^0
  Fqr : Outport  OutDataType=sfix(16)  OutScaling=2^0
  wires:
  wr/1 -> Add/2
  Add/1 -> 1/wb/1
  1/wb/1 -> Product/1
  Fdr/1 -> Product/2
  Product/1 -> Add1/1
  Add1/1 -> wb/1
  wb/1 -> Integrator/1
  Integrator/1 -> Fqr/1, Add2/2
  Fmq/1 -> Add2/1
  Add2/1 -> Rr/Xlr/1
  Rr/Xlr/1 -> Add1/2
  we/1 -> Add/1

== system IFOR/Asynchronmotormodell/Flussberechnung/Fqs1 ==
  Fds : Inport  OutDataType=sfix(16)  OutScaling=2^0
  Vqs : Inport  Port=2  OutDataType=sfix(16)  OutScaling=2^0
  Fmq : Inport  Port=3  OutDataType=sfix(16)  OutScaling=2^0
  we : Inport  Port=4  OutDataType=sfix(16)  OutScaling=2^0
  1/wb : Gain  Gain=1/wb  ParameterDataType=sfix(16)  ParameterScaling=2^0  OutDataType=sfix(16)  OutScaling=2^0
  Add1 : Sum  Inputs=+-+  OutDataType=sfix(16)  OutScaling=2^-10
  Add2 : Sum  Inputs=+-  OutDataType=sfix(16)  OutScaling=2^-10
  Integrator : Integrator
  Product : Product  OutDataType=sfix(16)  OutScaling=2^0  RndMeth=Zero
  Rs/Xls : Gain  Gain=Rs/Xls  ParameterDataType=sfix(16)  ParameterScaling=2^0  OutDataType=sfix(16)  OutScaling=2^0
  wb : Gain  Gain=wb  ParameterDataType=sfix(16)  ParameterScaling=2^0  OutDataType=sfix(16)  OutScaling=2^0
  Fqs : Outport  OutDataType=sfix(16)  OutScaling=2^0
  wires:
  we/1 -> 1/wb/1
  1/wb/1 -> Product/1
  Fds/1 -> Product/2
  Product/1 -> Add1/2
  Vqs/1 -> Add1/1
  Fmq/1 -> Add2/1
  Add2/1 -> Rs/Xls/1
  Rs/Xls/1 -> Add1/3
  Add1/1 -> wb/1
  wb/1 -> Integrator/1
  Integrator/1 -> Fqs/1, Add2/2
